simulink model "dpr_test"  (R2019b)
settings: Solver=FixedStepDiscrete  StartTime=0.0  StopTime=stopTime  RelTol=1e-3
InitFcn:
  | initCallback
StopFcn:
  | stopCallback
undefined symbols (not defined in the file or in its folder): config
libraries: hdlsllib x2
settings Model: SimulationMode=accelerator  Creator=Ross  LastModifiedBy=tyler
settings SolverCC: AutoInsertRateTranBlk=on
settings DataIOCC: ReturnWorkspaceOutputs=off
settings OptimizationCC: BlockReduction=off  ConditionallyExecuteInputs=off  DefaultParameterBehavior=Inlined
settings DebuggingCC: SignalInfNanChecking=error  SignalRangeChecking=warning  ReadBeforeWriteMsg=DisableAll  WriteAfterWriteMsg=DisableAll  WriteAfterReadMsg=DisableAll  AlgebraicLoopMsg=error  MultiTaskDSMMsg=none  SingleTaskRateTransMsg=error  ParameterUnderflowMsg=warning  UnderSpecifiedDataTypeMsg=error  PregeneratedLibrarySubsystemCodeDiagnostic=none  ArithmeticOperatorsInVariantConditions=warning
settings HardwareCC: ProdBitPerPointer=32  ProdBitPerSizeT=32  ProdBitPerPtrDiffT=32  ProdLargestAtomicFloat=None  ProdIntDivRoundTo=Undefined  ProdEndianess=Unspecified  ProdWordSize=32  ProdHWDeviceType=ASIC/FPGA->ASIC/FPGA  TargetBitPerPointer=64  TargetBitPerSizeT=64  TargetBitPerPtrDiffT=64  TargetLongLongMode=on  TargetIntDivRoundTo=Zero  TargetEndianess=LittleEndian  TargetWordSize=64  TargetHWDeviceType=Custom Processor->MATLAB Host Computer  ProdEqTarget=off
settings ModelReferenceCC: UpdateModelReferenceTargets=IfOutOfDate
settings SFSimCC: SFSimEcho=off  SimUseLocalCustomCode=off  CustomCodeUndefinedFunction=UseInterfaceOnly
settings RTWCC: RTWUseLocalCustomCode=off

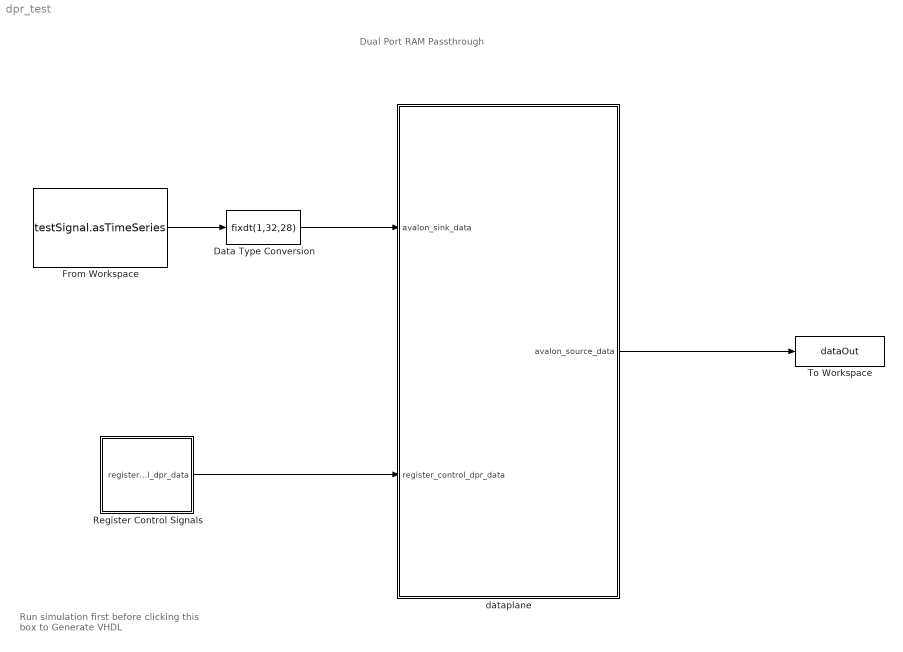
== system dpr_test ==
  note: Dual Port RAM Passthrough
  note: Run simulation first
      | before clicking this box to
      | Generate VHDL
  Data Type Conversion : DataTypeConversion  OutDataTypeStr=fixdt(1,32,28)
  From Workspace : FromWorkspace  VariableName=testSignal.asTimeSeries  OutDataTypeStr=double  SampleTime=1 / config.system.sampleClockFrequency  Interpolate=off  OutputAfterFinalValue=Setting to zero
  Register Control Signals : Subsystem
  To Workspace : ToWorkspace  VariableName=dataOut  SaveFormat=Timeseries  SampleTime=-1
      settings: Save2DSignal=2-D array (concatenate along first dimension)
  dataplane : Subsystem  TreatAsAtomicUnit=on
  wires:
  dataplane/1(avalon_source_data) -> To Workspace/1
  From Workspace/1 -> Data Type Conversion/1
  Data Type Conversion/1 -> dataplane/1(avalon_sink_data)
  Register Control Signals/1("register_control_dpr_data ") -> dataplane/2(register_control_dpr_data)

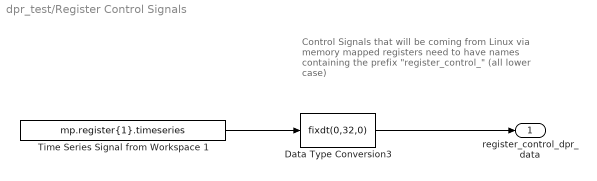
== system dpr_test/Register Control Signals ==
  note: Control Signals that will be coming from Linux via
      | memory mapped registers need to have names
      | containing the prefix "register_control_"
      | (all lower case)
  Data Type Conversion3 : DataTypeConversion  OutDataTypeStr=fixdt(0,32,0)
  Time Series Signal from Workspace 1 : FromWorkspace  VariableName=mp.register{1}.timeseries  OutDataTypeStr=double  SampleTime=1 / config.system.sampleClockFrequency
  "register_control_dpr_data " : Outport  VectorParamsAs1DForOutWhenUnconnected=off
  wires:
  Time Series Signal from Workspace 1/1 -> Data Type Conversion3/1
  Data Type Conversion3/1 -> "register_control_dpr_data "/1

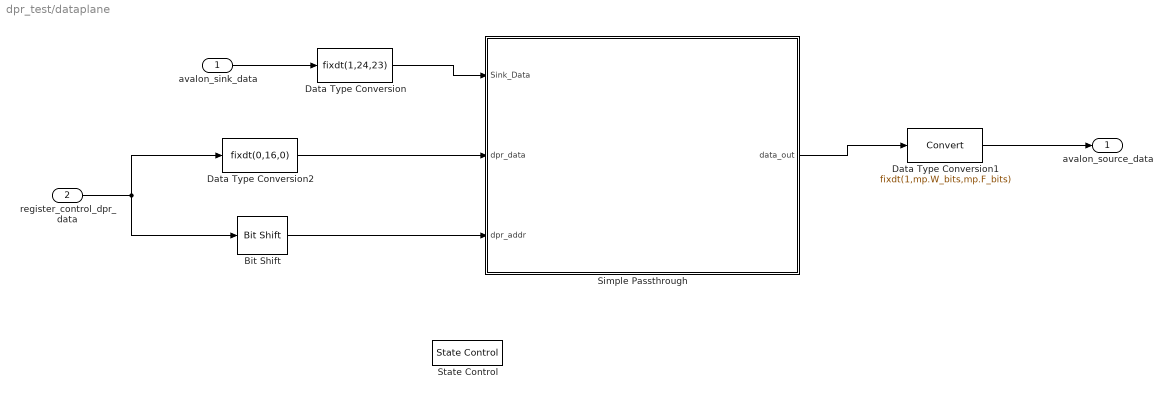
== system dpr_test/dataplane ==
  avalon_sink_data : Inport
  register_control_dpr_data : Inport  Port=2
  Bit Shift : hdlsllib/Logic and Bit Operations/Bit Shift  mode=Shift Right Logical  N=16
      settings: SourceProductName=Simulink
  Data Type Conversion : DataTypeConversion  OutDataTypeStr=fixdt(1,24,23)
  Data Type Conversion1 : DataTypeConversion  OutDataTypeStr=fixdt(1,mp.W_bits,mp.F_bits)
  Data Type Conversion2 : DataTypeConversion  OutDataTypeStr=fixdt(0,16,0)
  "Simple Passthrough " : Subsystem
  State Control : StateControl  StateControl=Synchronous
  avalon_source_data : Outport  VectorParamsAs1DForOutWhenUnconnected=off
  wires:
  Data Type Conversion1/1 -> avalon_source_data/1
  avalon_sink_data/1 -> Data Type Conversion/1
  "Simple Passthrough "/1(data_out) -> Data Type Conversion1/1
  Data Type Conversion/1 -> "Simple Passthrough "/1(Sink_Data)
  Data Type Conversion2/1 -> "Simple Passthrough "/2(dpr_data)
  Bit Shift/1 -> "Simple Passthrough "/3(dpr_addr)
  register_control_dpr_data/1 -> Data Type Conversion2/1, Bit Shift/1

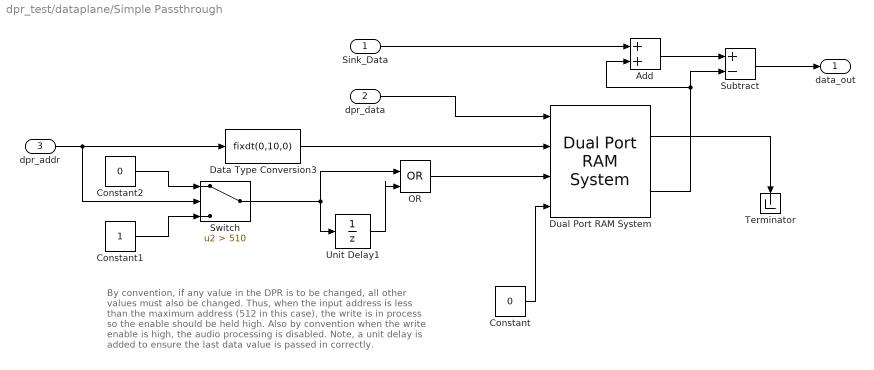
== system dpr_test/dataplane/Simple Passthrough  ==
  note: By convention, if any value in the DPR is to be changed, all other
      | values must also be changed.  Thus, when the input address is
      | less than the maximum address (512 in this case), the write is in
      | process so the enable should be held high.  Also by convention
      | when the write enable is high, the audio processing is disabled.
      | Note, a unit delay is added to ensure the last data value is passed
      | in correctly.
  Sink_Data : Inport
  dpr_data : Inport  Port=2
  dpr_addr : Inport  Port=3
  Add : Sum
  Constant : Constant  Value=0  OutDataTypeStr=fixdt(0,10,0)  SampleTime=-1
  Constant1 : Constant  OutDataTypeStr=boolean  SampleTime=-1
  Constant2 : Constant  Value=0  OutDataTypeStr=boolean  SampleTime=-1
  Data Type Conversion3 : DataTypeConversion  OutDataTypeStr=fixdt(0,10,0)
  Dual Port RAM System : hdlsllib/HDL RAMs/Dual Port RAM System  RAMType=Dual port  WriteOutputValue=New data  RAMInitialValue=0  SimulateUsing=Code generation
      settings: SourceProductName=Simulink  SourceProductBaseCode=SL
  OR : Logic  Operator=OR  IconShape=distinctive  AllPortsSameDT=off  OutDataTypeStr=boolean
  Subtract : Sum  Inputs=+-
  Switch : Switch  Criteria=u2 > Threshold  Threshold=510  OutDataTypeStr=boolean
  Terminator : Terminator
  Unit Delay1 : UnitDelay  SampleTime=-1  HasFrameUpgradeWarning=on
  data_out : Outport
  wires:
  dpr_data/1 -> Dual Port RAM System/1
  Constant/1 -> Dual Port RAM System/4
  Sink_Data/1 -> Add/1
  Add/1 -> Subtract/1
  Dual Port RAM System/2 -> Add/2, Subtract/2
  Subtract/1 -> data_out/1
  Dual Port RAM System/1 -> Terminator/1
  Data Type Conversion3/1 -> Dual Port RAM System/2
  dpr_addr/1 -> Data Type Conversion3/1, Switch/2
  OR/1 -> Dual Port RAM System/3
  Unit Delay1/1 -> OR/2
  Constant1/1 -> Switch/3
  Constant2/1 -> Switch/1
  Switch/1 -> OR/1, Unit Delay1/1
